simulink model "onephaseACVoltageControl"  (R2016b)
settings: Solver=VariableStepAuto  StartTime=0.0  StopTime=0.1  RelTol=1e-3
libraries: powerlib x9, dspstat3 x4
settings Model: Creator=lenovo  LastModifiedBy=lenovo

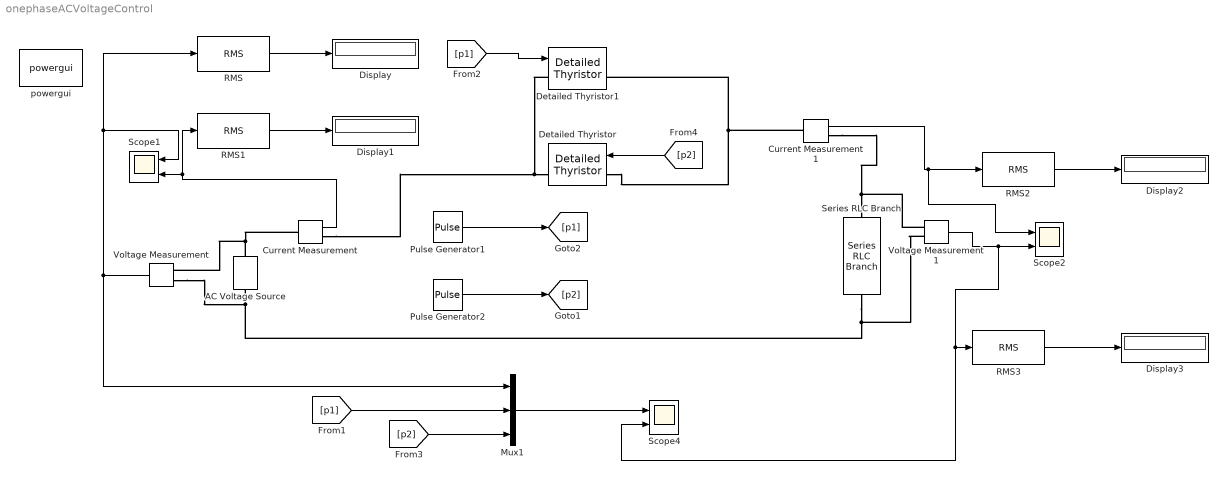
== system onephaseACVoltageControl ==
  AC Voltage Source : powerlib/Electrical Sources/AC Voltage Source  Amplitude=24*1.414  Phase=0  Frequency=50  SampleTime=0  Measurements=None  BusType=swing  Pref=10e3  Qref=0  Qmin=-inf  Qmax=+inf
  Current Measurement : powerlib/Measurements/Current Measurement  PhasorSimulation=off  OutputType=Complex  PSBequivalent=0
  Current Measurement1 : powerlib/Measurements/Current Measurement  PhasorSimulation=off  OutputType=Complex  PSBequivalent=0
  Detailed Thyristor : powerlib/Power Electronics/Detailed Thyristor  Ron=0.001  Lon=1e-3  Vf=0.8  IL=0.1  Tq=100e-6  IC=0  Rs=500  Cs=250e-9  Measurements=on
  Detailed Thyristor1 : powerlib/Power Electronics/Detailed Thyristor  Ron=0.001  Lon=1e-3  Vf=0.8  IL=0.1  Tq=100e-6  IC=0  Rs=500  Cs=250e-9  Measurements=on
  Display{,1..3} (4 alike) : Display
  Mux1 : Mux  Inputs=3
  Pulse Generator1 : DiscretePulseGenerator  PulseType=Time based  Amplitude=15  Period=1/50  PulseWidth=5  PhaseDelay=((1/50)/360)*90
  Pulse Generator2 : DiscretePulseGenerator  PulseType=Time based  Amplitude=15  Period=1/50  PulseWidth=5  PhaseDelay=(((1/50)/360)*90)+((1/50)/2)
  RMS{,1..3} (4 alike) : dspstat3/RMS  run=off  directionMode=Each column  dimension=1  InputProcessing=Columns as channels (frame based)  reset_popup=None
  Scope1 : Scope  NumInputPorts=2
  Scope2 : Scope  NumInputPorts=2
  Scope4 : Scope  NumInputPorts=2
  Series RLC Branch : powerlib/Elements/Series RLC Branch  LConnTagsString=__new0  RConnTagsString=__new0  BranchType=R  Resistance=100  Inductance=0.001  SetiL0=off  InitialCurrent=0  Capacitance=1e-6  Setx0=off  InitialVoltage=0  Measurements=None
  Voltage Measurement : powerlib/Measurements/Voltage Measurement  PhasorSimulation=off  OutputType=Complex  PSBequivalent=0
  Voltage Measurement1 : powerlib/Measurements/Voltage Measurement  PhasorSimulation=off  OutputType=Complex  PSBequivalent=0
  powergui : powerlib/powergui  Priority=1  SimulationMode=Continuous  SolverType=Tustin/Backward Euler (TBE)  SampleTime=50e-6  frequency=60  SPID=off  DisableSnubberDevices=off  DisableRonSwitches=off  DisableVfSwitches=off  SwTol=0  DisplayEquations=off  Interpol=off  ExternalGateDelay=off  methode=off  Ts=10  FunctionMessages=off  echomessages=off  HookPort=off  EnableUseOfTLC=off  x0status=blocks  frequencyindice=0  Pbase=100e6  ErrMax=1e-4  Iterations=50  UnitsV=kV  UnitsW=MW  buscounter=0  RestoreLinks=warning  ResistiveCurrentMeasurement=off  Frange=[0:2:500]  Ylog=off  Xlog=on  ShowGrid=off  save=off  variable=ZData  structure=0  ZoomFFT=off  StartTime=0.0  cycles=1  DisplayStyle=1  fundamental=60  FreqAxis=off  MaxFrequency=1000  frequencyindicesteady=1  RmsSteady=1  display=off
  wires:
  Voltage Measurement/1 -> Mux1/1, Scope1/1, RMS/1
  RMS1/1 -> Display1/1
  RMS/1 -> Display/1
  Current Measurement/1 -> Scope1/2, RMS1/1
  [p1] -> Mux1/2
  [p2] -> Mux1/3
  Mux1/1 -> Scope4/1
  Pulse Generator1/1 -> [p1]
  Pulse Generator2/1 -> [p2]
  [p1] -> Detailed Thyristor1/1
  [p2] -> Detailed Thyristor/1
  Current Measurement1/1 -> Scope2/1, RMS2/1
  RMS2/1 -> Display2/1
  Voltage Measurement1/1 -> Scope4/2, RMS3/1, Scope2/2
  RMS3/1 -> Display3/1
  connections:
  AC Voltage Source/RConn1 -- Current Measurement/LConn1 -- Voltage Measurement/LConn2
  Voltage Measurement/LConn1 -- Voltage Measurement1/LConn2 -- Series RLC Branch/RConn1 -- AC Voltage Source/LConn1
  Detailed Thyristor1/LConn1 -- Current Measurement/RConn1 -- Detailed Thyristor/RConn1
  Detailed Thyristor/LConn1 -- Current Measurement1/LConn1 -- Detailed Thyristor1/RConn1
  Current Measurement1/RConn1 -- Voltage Measurement1/LConn1 -- Series RLC Branch/LConn1
